simulink model "bldc_sixstep_f28069mLaunchPad"  (R2023b)
settings: Solver=FixedStepAuto  StartTime=0.0  StopTime=1.6  RelTol=1e-3  EnableMultiTasking=on
values from neighbouring files (symbols this model uses):
  bldc = mcb_SetPMSMMotorParameters('Teknic2310P')    [bldc_sixstep_f28069mLaunchPad_data.m]
  inverter = mcb_SetInverterParameters('BoostXL-DRV8305')    [bldc_sixstep_f28069mLaunchPad_data.m]
  PI_params = mcb_SetControllerParameters(bldc,inverter,PU_System,T_pwm,2*Ts,Ts_speed)    [bldc_sixstep_f28069mLaunchPad_data.m]
  PWM_frequency = 20e3    (= 20000)    [bldc_sixstep_f28069mLaunchPad_data.m]
  target = mcb_SetProcessorDetails('F28069M',PWM_frequency)    [bldc_sixstep_f28069mLaunchPad_data.m]
  Ts = T_pwm    (= 5e-05)    [bldc_sixstep_f28069mLaunchPad_data.m]
  Ts_motor_simscape = T_pwm/100    (= 5e-07)    [bldc_sixstep_f28069mLaunchPad_data.m]
  Ts_simulink = T_pwm/2    (= 2.5e-05)    [bldc_sixstep_f28069mLaunchPad_data.m]
  Ts_speed = 10*Ts    (= 0.0005)    [bldc_sixstep_f28069mLaunchPad_data.m]
libraries: nesl_utility x14, fl_lib x9, pil_lib x6, mcbcontrolslib x5, simulink x5, ee_lib x5, slpidlib x3, mcbpositiondecoderlib x2
(part 2 of 2)

== system bldc_sixstep_f28069mLaunchPad/Controller/Speed Control1/PI_Controller_Speed ==
  N_ref : Inport
  N_fb : Inport  Port=2
  Constant : Constant
  Discrete PI Controller with anti-windup & reset : slpidlib/PID Controller  Controller=PI  Form=Parallel  TimeDomain=Discrete-time  UseExternalTs=off  SampleTime=-1  IntegratorMethod=Forward Euler  FilterMethod=Forward Euler  ControllerParametersSource=external  P=1  I=1  UseKiTs=on  D=0  N=100  UseFilter=on  TunerSelectOption=Transfer Function Based (PID Tuner App)  InitialConditionSource=external  InitialConditionForIntegrator=0  InitialConditionForFilter=0  DifferentiatorICPrevScaledInput=0  ExternalReset=level  TrackingMode=off  Kt=1  LimitOutput=on  SatLimitsSource=internal  UpperSaturationLimit=1  LowerSaturationLimit=-1  LinearizeAsGain=on  AntiWindupMode=clamping  Kb=1  LimitIntegrator=off  UpperIntegratorSaturationLimit=inf  LowerIntegratorSaturationLimit=-inf  RndMeth=Simplest  POutMin=[]  POutMax=[]  IOutMin=[]  IOutMax=[]  DOutMin=[]  DOutMax=[]  NOutMin=[]  NOutMax=[]  SumOutMin=[]  SumOutMax=[]  SaturationOutDataTypeStr=Inherit: Inherit via back propagation  SaturationOutMin=[]  SaturationOutMax=[]  PParamMin=[]  PParamMax=[]  IParamMin=[]  IParamMax=[]  DParamMin=[]  DParamMax=[]  NParamMin=[]  NParamMax=[]  KbParamMin=[]  KbParamMax=[]  KtParamMin=[]  KtParamMax=[]  KbOutMin=[]  KbOutMax=[]  KtOutMin=[]  KtOutMax=[]  IntegratorOutMin=[]  IntegratorOutMax=[]  FilterOutMin=[]  FilterOutMax=[]  SumI1OutMin=[]  SumI1OutMax=[]  SumI2OutMin=[]  SumI2OutMax=[]  SumI3OutMin=[]  SumI3OutMax=[]  SumI4OutMin=[]  SumI4OutMax=[]  SumDOutMin=[]  SumDOutMax=[]  DifferentiatorOutMin=[]  DifferentiatorOutMax=[]  FilterDiffOutCoefMin=[]  FilterDiffOutCoefMax=[]  ReciprocalOutMin=[]  ReciprocalOutMax=[]  SumDenOutMin=[]  SumDenOutMax=[]  SumNumOutMin=[]  SumNumOutMax=[]  DivideOutMin=[]  DivideOutMax=[]  UdiffTsProdOutMin=[]  UdiffTsProdOutMax=[]  NTsProdOutMin=[]  NTsProdOutMax=[]  UintegralTsProdOutMin=[]  UintegralTsProdOutMax=[]  UngainTsProdOutMin=[]  UngainTsProdOutMax=[]  ClampingZeroOutDataTypeStr=Inherit: Inherit via back propagation  ClampingZeroOutMin=[]  ClampingZeroOutMax=[]  FilterDenConstantOutDataTypeStr=Inherit: Inherit via back propagation  FilterDenConstantOutMin=[]  FilterDenConstantOutMax=[]  PCopyOutDataTypeStr=Inherit: Inherit via back propagation  PCopyOutMin=[]  PCopyOutMax=[]  NCopyOutDataTypeStr=Inherit: Inherit via back propagation  NCopyOutMin=[]  NCopyOutMax=[]  IntegratorContinuousStateAttributes=''  IntegratorStateMustResolveToSignalObject=off  IntegratorRTWStateStorageClass=Auto  FilterContinuousStateAttributes=''  FilterStateMustResolveToSignalObject=off  FilterRTWStateStorageClass=Auto  ParallelPVariant=ExternalParameters  IdealPVariant=Disabled  IVariant=ExternalParameters  DVariant=Disabled  IntegratorVariant=Discrete  SatVariant=Enabled  AWVariant=DiscClampingParallel  PCopyVariant=Disabled  TRVariant=Disabled  FdbkBlocksVariant=Forward  IdealPFdbkVariant=Disabled  SatFdbkVariant=Disabled  DerivativeFilterVariant=Disabled  NVariant=Disabled  NCopyVariant=Disabled_SignalSpec  FilterICVariant=Disabled  IntegratorICVariant=ExternalICs  ExternalResetVariant=ExternalReset  TRSumVariant=Passthrough  SumFdbkVariant=Disabled  SumVariant=Sum_PI  TsampFilterVariant=InternalTs  TsampNgainVariant=Passthrough  TsampIntegralVariant=Disabled_SignalSpec  ExternalSaturationOutDataTypeStr=Inherit: Same as second input
      settings: LibrarySourceBlock=mcbcontrolslib/PI Controller
  Ki1 : Constant  Value=PI_params.Ki_speed*Ts_speed  OutDataTypeStr=dataType  SampleTime=-1
  Ki2 : Constant  Value=0  OutDataTypeStr=dataType  SampleTime=-1
  Kp1 : Constant  Value=PI_params.Kp_speed  OutDataTypeStr=dataType  SampleTime=-1
  Logical Operator : Logic  Operator=NOT  IconShape=distinctive  AllPortsSameDT=off  OutDataTypeStr=boolean
  Sum : Sum  Inputs=|+-  RndMeth=Round
  Zero_Cancellation : mcbcontrolslib/IIR Filter  VariantControl=Low Pass Filter  VariantSelect=Low-pass  Filter_constant=0.01*(Ts_speed/Ts)  advancedSettings=off  Ts=50e-6  cutOff_freq=353.6777
  Idc_ref : Outport  VectorParamsAs1DForOutWhenUnconnected=off
  wires:
  Discrete PI Controller with anti-windup & reset/1 -> Idc_ref/1
  Ki1/1 -> Discrete PI Controller with anti-windup & reset/3
  Kp1/1 -> Discrete PI Controller with anti-windup & reset/2
  N_fb/1 -> Sum/2
  N_ref/1 -> Zero_Cancellation/1
  Logical Operator/1 -> Discrete PI Controller with anti-windup & reset/4
  Ki2/1 -> Discrete PI Controller with anti-windup & reset/5
  Sum/1 -> Discrete PI Controller with anti-windup & reset/1
  Constant/1 -> Logical Operator/1
  Zero_Cancellation/1 -> Sum/1

== system bldc_sixstep_f28069mLaunchPad/Controller/Speed Control1/Speed_Ref_Selector ==
  Speed_Ref_In : Inport
  Speed_Ref_Open : Inport  Port=2
  Constant : Constant
  Switch : Switch  Criteria=u2 > Threshold  Threshold=0.5  SaturateOnIntegerOverflow=off  InputSameDT=off
  Speed_Ref_PU : Outport
  wires:
  Switch/1 -> Speed_Ref_PU/1
  Constant/1 -> Switch/2
  Speed_Ref_Open/1 -> Switch/3
  Speed_Ref_In/1 -> Switch/1

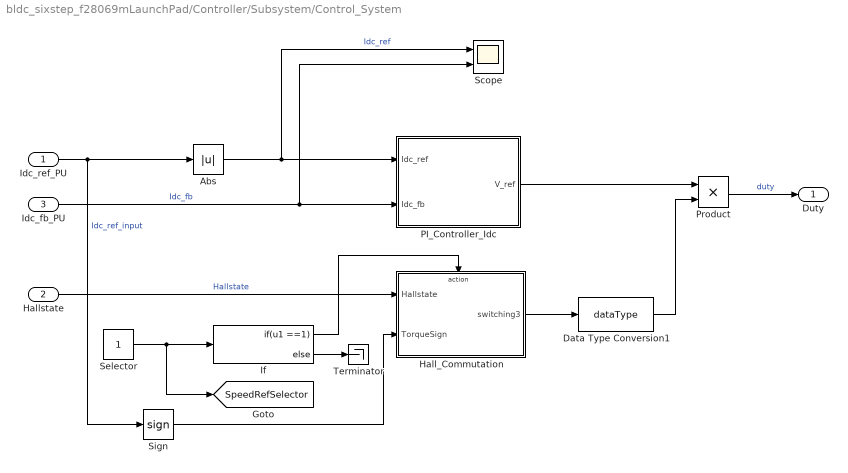
== system bldc_sixstep_f28069mLaunchPad/Controller/Subsystem/Control_System ==
  Idc_ref_PU : Inport
  Hallstate : Inport  Port=2
  Idc_fb_PU : Inport  Port=3
  Abs : Abs  SaturateOnIntegerOverflow=off
  Data Type Conversion1 : DataTypeConversion  OutDataTypeStr=dataType  RndMeth=Simplest  SaturateOnIntegerOverflow=off
  Hall_Commutation : Subsystem
  If : If  IfExpression=u1 ==1
  PI_Controller_Idc : Subsystem
  Product : Product  RndMeth=Simplest  OutDataTypeStr=Inherit: Same as first input
  Scope : Scope  NumInputPorts=2
  Selector : Constant  OutDataTypeStr=uint16  SampleTime=-1
  Sign : Signum
  Terminator : Terminator
  Duty : Outport  VectorParamsAs1DForOutWhenUnconnected=off
  tag scope: SpeedRefSelector=global
  wires:
  Hallstate/1 -> Hall_Commutation/1(Hallstate)  "Hallstate"
  If/1 -> Hall_Commutation/Action
  Idc_fb_PU/1 -> Scope/2, PI_Controller_Idc/2(Idc_fb)  "Idc_fb"
  Abs/1 -> Scope/1, PI_Controller_Idc/1(Idc_ref)  "Idc_ref"
  PI_Controller_Idc/1(V_ref) -> Product/1
  Idc_ref_PU/1 -> Sign/1, Abs/1  "Idc_ref_input"
  Product/1 -> Duty/1  "duty"
  Selector/1 -> If/1, [SpeedRefSelector]
  Sign/1 -> Hall_Commutation/2(TorqueSign)
  Data Type Conversion1/1 -> Product/2
  Hall_Commutation/1(switching3) -> Data Type Conversion1/1
  If/2 -> Terminator/1

== system bldc_sixstep_f28069mLaunchPad/Controller/Subsystem/Input scaling ==
  Iabc_meas_ADC : Inport
  Hall_Meas : Inport  Port=2
  Convert ADC value to PU : Subsystem
  Hall Feedback : Subsystem  TreatAsAtomicUnit=on
  Hall selected : Constant
  If : If  IfExpression=u1 ==1
  Terminator : Terminator
  Terminator1 : Terminator
  speed_PU : Outport  InitialOutput=0  VectorParamsAs1DForOutWhenUnconnected=off
  HallState : Outport  Port=2  InitialOutput=0  VectorParamsAs1DForOutWhenUnconnected=off
  Idc_meas_PU : Outport  Port=3
  wires:
  Hall Feedback/1(HallState) -> HallState/1
  Hall_Meas/1 -> Hall Feedback/1(Hall_Meas)
  If/1 -> Hall Feedback/Action
  Hall selected/1 -> If/1
  Hall Feedback/2(Speed_PU) -> speed_PU/1
  If/2 -> Terminator/1
  Iabc_meas_ADC/1 -> Convert ADC value to PU/1(Iabc_meas_ADC)
  Convert ADC value to PU/1(Idc_meas_PU) -> Idc_meas_PU/1
  Convert ADC value to PU/2(Ia_meas_PU) -> Terminator1/1

== system bldc_sixstep_f28069mLaunchPad/Controller/Subsystem/Inverter ==
  Inverter Signals : Inport
  Constant : Constant
  Data Type Duplicate : DataTypeDuplicate
  Switch : Switch  Threshold=0.5  RndMeth=Simplest  SaturateOnIntegerOverflow=off  InputSameDT=off
  stop : Constant  Value=[0 0 0 0 0 0]  OutDataTypeStr=Inherit: Inherit via back propagation
  Duty : Outport  VectorParamsAs1DForOutWhenUnconnected=off
  wires:
  Constant/1 -> Switch/2
  Switch/1 -> Duty/1
  Inverter Signals/1 -> Switch/1, Data Type Duplicate/1  "PWM Duty Cycles"
  stop/1 -> Switch/3, Data Type Duplicate/2

== system bldc_sixstep_f28069mLaunchPad/Controller/Subsystem/Sensor Driver Block ==
  fb_sim : Inport
  Bus Selector : BusSelector  OutputSignals=Iabc_fb,Hall_fb
  Iabc_Meas_ADC : Outport
  Hall_Meas : Outport  Port=2
  wires:
  Bus Selector/1 -> Iabc_Meas_ADC/1  "<Iabc_fb>"
  fb_sim/1 -> Bus Selector/1
  Bus Selector/2 -> Hall_Meas/1  "<Hall_fb>"

== system bldc_sixstep_f28069mLaunchPad/Controller - SIL/Subsystem/__InputSSForSFun__ ==
  Speed_ref_PU : Inport
  fb_sim : Inport  Port=2
  temporaryBusSelectName_1 : BusSelector  OutputSignals=Iabc_fb,Hall_fb
  __UniqueOutportName__1__ : Outport
  __UniqueOutportName__2__ : Outport  Port=2
  __UniqueOutportName__3__ : Outport  Port=3
  wires:
  temporaryBusSelectName_1/2 -> __UniqueOutportName__3__/1  "<Hall_fb>"
  temporaryBusSelectName_1/1 -> __UniqueOutportName__2__/1  "<Iabc_fb>"
  Speed_ref_PU/1 -> __UniqueOutportName__1__/1
  fb_sim/1 -> temporaryBusSelectName_1/1

== system bldc_sixstep_f28069mLaunchPad/Controller - SIL/Subsystem/__OutputSSForSFun__ ==
  __UniqueInportName__1__ : Inport
  Duty cycles : Outport
  wires:
  __UniqueInportName__1__/1 -> Duty cycles/1

== system bldc_sixstep_f28069mLaunchPad/Current control - SIL/Current control - SIL/__InputSSForSFun__ ==
  Idc_ref_PU : Inport
  fb_sim : Inport  Port=2
  temporaryBusSelectName_1 : BusSelector  OutputSignals=Iabc_fb,Hall_fb
  __UniqueOutportName__1__ : Outport
  __UniqueOutportName__2__ : Outport  Port=2
  __UniqueOutportName__3__ : Outport  Port=3
  wires:
  temporaryBusSelectName_1/2 -> __UniqueOutportName__3__/1  "<Hall_fb>"
  temporaryBusSelectName_1/1 -> __UniqueOutportName__2__/1  "<Iabc_fb>"
  Idc_ref_PU/1 -> __UniqueOutportName__1__/1
  fb_sim/1 -> temporaryBusSelectName_1/1

== system bldc_sixstep_f28069mLaunchPad/Current control - SIL/Current control - SIL/__OutputSSForSFun__ ==
  __UniqueInportName__1__ : Inport
  __UniqueInportName__2__ : Inport  Port=2
  Duty cycles : Outport
  Speed_fb_PU : Outport  Port=2
  wires:
  __UniqueInportName__2__/1 -> Speed_fb_PU/1
  __UniqueInportName__1__/1 -> Duty cycles/1

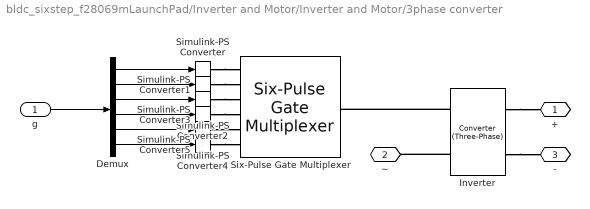
== system bldc_sixstep_f28069mLaunchPad/Inverter and Motor/Inverter and Motor/3phase converter ==
  g : Inport
  Demux : Demux  Outputs=6
  Inverter : ee_lib/Semiconductors & Converters/Converters/Converter (Three-Phase)  port_option=ee.enum.threePhasePort.composite  device_type=ee.enum.converters.switchingdevice.mosfet  K=0  Vf=0.8 V  Ron=0.001 Ohm  Rds=inverter.Rds_on Ohm  Goff=1e-5 1/Ohm  Vgt=1 V  Vgt_off=-1 V  Ih=1 A  Vth=0.7 V  diode_param=ee.enum.converters.protectiondiode.nodynamics  diode_Vf=0.7 V  diode_Ron=inverter.Rds_on Ohm  diode_Goff=1e-5 1/Ohm  diode_C=50 nF  diode_iRM=-235 A  diode_iF=300 A  diode_idot=-50 A/us  diode_trr_param=ee.enum.converters.diodetrr.trr_factor  diode_trr_factor=3  diode_trr=15 us  diode_Qrr=1.5e+3 s*uA  snubber_type=ee.enum.converters.snubber.exclude  Cs=1e-7 F  Rs=0.1 Ohm
  Simulink-PS Converter{,1..5} (6 alike) : nesl_utility/Simulink-PS Converter  PhysicalDomain=network_engine_domain  SubClassName=ps_input  LeftPortType=input  RightPortType=output  PseudoPeriodic=off  Frequencies=[]  NoiseDistribution=none  NoiseParameters=[]  Unit=1  AffineConversion=off  FilteringAndDerivatives=provide  SimscapeFilterOrder=1  InputFilterTimeConstant=0.001  UdotUserProvided=0
  Six-Pulse Gate Multiplexer : ee_lib/Semiconductors & Converters/Converters/Six-Pulse Gate Multiplexer  port_option=ee.enum.controlport.ps
  + : PMIOPort  Side=Right
  ~ : PMIOPort  Port=2  Side=Left
  - : PMIOPort  Port=3  Side=Right
  wires:
  g/1 -> Demux/1
  Demux/1 -> Simulink-PS Converter/1
  Demux/2 -> Simulink-PS Converter1/1
  Demux/3 -> Simulink-PS Converter2/1
  Demux/4 -> Simulink-PS Converter3/1
  Demux/6 -> Simulink-PS Converter5/1
  Demux/5 -> Simulink-PS Converter4/1
  connections:
  Simulink-PS Converter/RConn1 -- Six-Pulse Gate Multiplexer/LConn1
  Inverter/RConn2 -- -/RConn1
  Inverter/RConn1 -- +/RConn1
  Inverter/LConn2 -- ~/RConn1
  Inverter/LConn1 -- Six-Pulse Gate Multiplexer/RConn1
  Simulink-PS Converter1/RConn1 -- Six-Pulse Gate Multiplexer/LConn2
  Simulink-PS Converter2/RConn1 -- Six-Pulse Gate Multiplexer/LConn3
  Simulink-PS Converter3/RConn1 -- Six-Pulse Gate Multiplexer/LConn4
  Simulink-PS Converter4/RConn1 -- Six-Pulse Gate Multiplexer/LConn5
  Simulink-PS Converter5/RConn1 -- Six-Pulse Gate Multiplexer/LConn6

== system bldc_sixstep_f28069mLaunchPad/Inverter and Motor/Inverter and Motor/6-pulse PWM generator ==
  ModWave : Inport
  Relay : Relay
  Repeating Sequence Interpolated : simulink/Sources/Repeating Sequence Interpolated  OutValues="[0 1   0].'"  TimeValues=0.25/fs*[0 2 4].'  LookUpMeth=Interpolation-Use End Values  tsamp=Ts_motor_simscape  OutMin=[]  OutMax=[]  OutDataTypeStr=double  OutputDataTypeScalingMode=double  OutDataType=fixdt(0,8)  OutScaling=2^-10
  Sum : Sum  Inputs=|+-
  g : Outport
  wires:
  Relay/1 -> g/1
  Repeating Sequence Interpolated/1 -> Sum/2  "carrier"
  Sum/1 -> Relay/1
  ModWave/1 -> Sum/1

== system bldc_sixstep_f28069mLaunchPad/Inverter and Motor/Inverter and Motor/Scale ==
  duty_abc : Inport
  Constant : Constant  Value=0  OutDataTypeStr=single  SampleTime=Ts_motor_simscape
  Data Type Conversion : DataTypeConversion  SaturateOnIntegerOverflow=off  RndMeth=Floor
  Gain : Gain
  Rate Transition : RateTransition
  Sum : Sum  Inputs=|++
  ModWave : Outport
  wires:
  Gain/1 -> Data Type Conversion/1
  Data Type Conversion/1 -> Rate Transition/1
  Rate Transition/1 -> ModWave/1  "ModWave"
  duty_abc/1 -> Sum/1  "beforeGain"
  Constant/1 -> Sum/2
  Sum/1 -> Gain/1

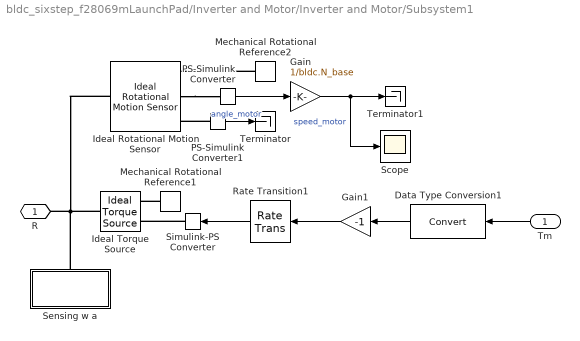
== system bldc_sixstep_f28069mLaunchPad/Inverter and Motor/Inverter and Motor/Subsystem1 ==
  Tm : Inport
  Data Type Conversion1 : DataTypeConversion  SaturateOnIntegerOverflow=off  RndMeth=Floor
  Gain : Gain  Gain=1/bldc.N_base
  Gain1 : Gain  Gain=-1
  Ideal Rotational Motion Sensor : fl_lib/Mechanical/Mechanical Sensors/Ideal Rotational Motion Sensor  reference=foundation.enum.MeasurementReference.difference  acceleration_port=false  velocity_port=true  position_port=true  wrap_angle=simscape.enum.onoff.off  offset=0 rad
  Ideal Torque Source : fl_lib/Mechanical/Mechanical Sources/Ideal Torque Source
  Mechanical Rotational Reference1 : fl_lib/Mechanical/Rotational Elements/Mechanical Rotational Reference
  Mechanical Rotational Reference2 : fl_lib/Mechanical/Rotational Elements/Mechanical Rotational Reference
  PS-Simulink Converter : nesl_utility/PS-Simulink Converter  PhysicalDomain=network_engine_domain  SubClassName=ps_output  LeftPortType=input  RightPortType=output  PseudoPeriodic=off  Frequencies=[]  VectorFormat=1-D array  Unit=rpm  AffineConversion=off
  PS-Simulink Converter1 : nesl_utility/PS-Simulink Converter  PhysicalDomain=network_engine_domain  SubClassName=ps_output  LeftPortType=input  RightPortType=output  PseudoPeriodic=off  Frequencies=[]  VectorFormat=1-D array  Unit=inherit  AffineConversion=off
  Rate Transition1 : RateTransition
  Scope : Scope
  Sensing w a : Subsystem
      mask Display: disp('w,Hall')
  Simulink-PS Converter : nesl_utility/Simulink-PS Converter  PhysicalDomain=network_engine_domain  SubClassName=ps_input  LeftPortType=input  RightPortType=output  PseudoPeriodic=off  Frequencies=[]  NoiseDistribution=none  NoiseParameters=[]  Unit=N*m  AffineConversion=off  FilteringAndDerivatives=provide  SimscapeFilterOrder=1  InputFilterTimeConstant=0.001  UdotUserProvided=0
  Terminator : Terminator
  Terminator1 : Terminator
  "R " : PMIOPort  Side=Right
  wires:
  Gain1/1 -> Rate Transition1/1
  Rate Transition1/1 -> Simulink-PS Converter/1
  Data Type Conversion1/1 -> Gain1/1
  Tm/1 -> Data Type Conversion1/1
  PS-Simulink Converter/1 -> Gain/1
  Gain/1 -> Scope/1, Terminator1/1  "speed_motor"
  PS-Simulink Converter1/1 -> Terminator/1  "angle_motor"
  connections:
  Mechanical Rotational Reference1/LConn1 -- Ideal Torque Source/RConn2
  Simulink-PS Converter/RConn1 -- Ideal Torque Source/RConn1
  Ideal Torque Source/LConn1 -- Sensing w a/LConn1 -- Ideal Rotational Motion Sensor/LConn1 -- "R "/RConn1
  Ideal Rotational Motion Sensor/RConn2 -- PS-Simulink Converter/LConn1
  PS-Simulink Converter1/LConn1 -- Ideal Rotational Motion Sensor/RConn3
  Mechanical Rotational Reference2/LConn1 -- Ideal Rotational Motion Sensor/RConn1

== system bldc_sixstep_f28069mLaunchPad/Inverter and Motor/Inverter and Motor/measVI ==
  Current Sensor (Three-Phase) : ee_lib/Sensors & Transducers/Current Sensor (Three-Phase)
  Line Voltage Sensor (Three-Phase) : ee_lib/Sensors & Transducers/Line Voltage Sensor (Three-Phase)
  PS-Simulink Converter2 : nesl_utility/PS-Simulink Converter  PhysicalDomain=network_engine_domain  SubClassName=ps_output  LeftPortType=input  RightPortType=output  PseudoPeriodic=off  Frequencies=[]  VectorFormat=1-D array  Unit=inherit  AffineConversion=off
  PS-Simulink Converter3 : nesl_utility/PS-Simulink Converter  PhysicalDomain=network_engine_domain  SubClassName=ps_output  LeftPortType=input  RightPortType=output  PseudoPeriodic=off  Frequencies=[]  VectorFormat=1-D array  Unit=inherit  AffineConversion=off
  ~1 From Inverter : PMIOPort  Side=Left
  ~2 to Motor : PMIOPort  Port=2  Side=Right
  tag scope: Iabc=global, Vabc=global
  wires:
  PS-Simulink Converter2/1 -> [Vabc]  "Vabc"
  PS-Simulink Converter3/1 -> [Iabc]  "Iabc"
  connections:
  Current Sensor (Three-Phase)/RConn1 -- PS-Simulink Converter3/LConn1
  PS-Simulink Converter2/LConn1 -- Line Voltage Sensor (Three-Phase)/RConn1
  Current Sensor (Three-Phase)/RConn2 -- ~2 to Motor/RConn1
  Line Voltage Sensor (Three-Phase)/LConn1 -- ~1 From Inverter/RConn1 -- Current Sensor (Three-Phase)/LConn1

== system bldc_sixstep_f28069mLaunchPad/Inverter and Motor/Sensor_Measurements/Halls ==
  x : Inport
  Demux : Demux  Outputs=3
  Gain : Gain  Gain=[4 2 1]  Multiplication=Matrix(K*u)
  Hall Signals HW : Subsystem
  Hall State Plant to HW : Subsystem
  Scope : Scope
  Scope1 : Scope  NumInputPorts=3
  Sum of Elements : Sum  Inputs=+
  y : Outport  VectorParamsAs1DForOutWhenUnconnected=off
  wires:
  Gain/1 -> Sum of Elements/1
  x/1 -> Gain/1
  Sum of Elements/1 -> Hall State Plant to HW/1(HallStatePlant)
  Hall State Plant to HW/1(HallstateHw) -> Scope/1, Hall Signals HW/1(HallState)  "HallState"
  Hall Signals HW/1(Hall Signals) -> Demux/1, y/1
  Demux/1 -> Scope1/1
  Demux/2 -> Scope1/2
  Demux/3 -> Scope1/3

== system bldc_sixstep_f28069mLaunchPad/Inverter and Motor/Sensor_Measurements/LowerSwitchCurrents ==
  In1 : Inport
  Constant : Constant  Value=0
  Switch : Switch  Criteria=u2 > Threshold  SaturateOnIntegerOverflow=off  InputSameDT=off
  cu : Outport
  wires:
  Constant/1 -> Switch/1
  In1/1 -> Switch/2, Switch/3
  Switch/1 -> cu/1  "cu"

== system bldc_sixstep_f28069mLaunchPad/Subsystem/Controller1/__InputSSForSFun__ ==
  Speed_ref : Inport
  fb_sim : Inport  Port=2
  temporaryBusSelectName_1 : BusSelector  OutputSignals=Iabc_fb,Hall_fb
  __UniqueOutportName__1__ : Outport
  __UniqueOutportName__2__ : Outport  Port=2
  __UniqueOutportName__3__ : Outport  Port=3
  wires:
  temporaryBusSelectName_1/2 -> __UniqueOutportName__3__/1  "<Hall_fb>"
  temporaryBusSelectName_1/1 -> __UniqueOutportName__2__/1  "<Iabc_fb>"
  Speed_ref/1 -> __UniqueOutportName__1__/1
  fb_sim/1 -> temporaryBusSelectName_1/1

== system bldc_sixstep_f28069mLaunchPad/Subsystem/Controller1/__OutputSSForSFun__ ==
  __UniqueInportName__1__ : Inport
  __UniqueInportName__2__ : Inport  Port=2
  __UniqueInportName__3__ : Inport  Port=3
  __UniqueInportName__4__ : Inport  Port=4
  __UniqueInportName__5__ : Inport  Port=5
  Speed ref : Outport
  Speed fb : Outport  Port=2
  Duty cycles : Outport  Port=3
  Idc ref : Outport  Port=4
  Idc_fb : Outport  Port=5
  wires:
  __UniqueInportName__5__/1 -> Idc_fb/1  "IDC"
  __UniqueInportName__4__/1 -> Idc ref/1
  __UniqueInportName__3__/1 -> Duty cycles/1
  __UniqueInportName__2__/1 -> Speed fb/1
  __UniqueInportName__1__/1 -> Speed ref/1

== system bldc_sixstep_f28069mLaunchPad/Controller/Subsystem/Control_System/Hall_Commutation ==
  Hallstate : Inport
  TorqueSign : Inport  Port=2
  Action Port : ActionPort  ActionPortLabel=if(u1 ==1)
  Six Step Commutation : mcbcontrolslib/Six Step Commutation  InputType=Hall  PositionUnit=Per unit  CommutationMode=120 deg  SequencePos=bldc.HallSequence  EnableCustomSwitching=off  CommutationSeqPos=[0 0 1 0 0 1;1 0 0 0 0 1;1 0 0 1 0 0;0 0 0 1 1 0;0 1 0 0 1 0;0 1 1 0 0 0]  CommutationSeqNeg="[0  1  1  0  0  0;0  1  0  0  1  0;0  0  0  1  1  0;1  0  0  1  0  0;1  0  0  0  0  1;0  0  1  0  0  1;]"
  switching3 : Outport
  wires:
  Hallstate/1 -> Six Step Commutation/1
  Six Step Commutation/1 -> switching3/1  "switching"
  TorqueSign/1 -> Six Step Commutation/2

== system bldc_sixstep_f28069mLaunchPad/Controller/Subsystem/Control_System/PI_Controller_Idc ==
  Idc_ref : Inport
  Idc_fb : Inport  Port=2
  Constant : Constant
  Discrete PI Controller with anti-windup & reset : slpidlib/PID Controller  Controller=PI  Form=Parallel  TimeDomain=Discrete-time  UseExternalTs=off  SampleTime=-1  IntegratorMethod=Forward Euler  FilterMethod=Forward Euler  ControllerParametersSource=external  P=1  I=1  UseKiTs=on  D=0  N=100  UseFilter=on  TunerSelectOption=Transfer Function Based (PID Tuner App)  InitialConditionSource=external  InitialConditionForIntegrator=0  InitialConditionForFilter=0  DifferentiatorICPrevScaledInput=0  ExternalReset=level  TrackingMode=off  Kt=1  LimitOutput=on  SatLimitsSource=internal  UpperSaturationLimit=1  LowerSaturationLimit=0  LinearizeAsGain=on  AntiWindupMode=clamping  Kb=1  LimitIntegrator=off  UpperIntegratorSaturationLimit=inf  LowerIntegratorSaturationLimit=-inf  RndMeth=Simplest  POutMin=[]  POutMax=[]  IOutMin=[]  IOutMax=[]  DOutMin=[]  DOutMax=[]  NOutMin=[]  NOutMax=[]  SumOutMin=[]  SumOutMax=[]  SaturationOutDataTypeStr=Inherit: Inherit via back propagation  SaturationOutMin=[]  SaturationOutMax=[]  PParamMin=[]  PParamMax=[]  IParamMin=[]  IParamMax=[]  DParamMin=[]  DParamMax=[]  NParamMin=[]  NParamMax=[]  KbParamMin=[]  KbParamMax=[]  KtParamMin=[]  KtParamMax=[]  KbOutMin=[]  KbOutMax=[]  KtOutMin=[]  KtOutMax=[]  IntegratorOutMin=[]  IntegratorOutMax=[]  FilterOutMin=[]  FilterOutMax=[]  SumI1OutMin=[]  SumI1OutMax=[]  SumI2OutMin=[]  SumI2OutMax=[]  SumI3OutMin=[]  SumI3OutMax=[]  SumI4OutMin=[]  SumI4OutMax=[]  SumDOutMin=[]  SumDOutMax=[]  DifferentiatorOutMin=[]  DifferentiatorOutMax=[]  FilterDiffOutCoefMin=[]  FilterDiffOutCoefMax=[]  ReciprocalOutMin=[]  ReciprocalOutMax=[]  SumDenOutMin=[]  SumDenOutMax=[]  SumNumOutMin=[]  SumNumOutMax=[]  DivideOutMin=[]  DivideOutMax=[]  UdiffTsProdOutMin=[]  UdiffTsProdOutMax=[]  NTsProdOutMin=[]  NTsProdOutMax=[]  UintegralTsProdOutMin=[]  UintegralTsProdOutMax=[]  UngainTsProdOutMin=[]  UngainTsProdOutMax=[]  ClampingZeroOutDataTypeStr=Inherit: Inherit via back propagation  ClampingZeroOutMin=[]  ClampingZeroOutMax=[]  FilterDenConstantOutDataTypeStr=Inherit: Inherit via back propagation  FilterDenConstantOutMin=[]  FilterDenConstantOutMax=[]  PCopyOutDataTypeStr=Inherit: Inherit via back propagation  PCopyOutMin=[]  PCopyOutMax=[]  NCopyOutDataTypeStr=Inherit: Inherit via back propagation  NCopyOutMin=[]  NCopyOutMax=[]  IntegratorContinuousStateAttributes=''  IntegratorStateMustResolveToSignalObject=off  IntegratorRTWStateStorageClass=Auto  FilterContinuousStateAttributes=''  FilterStateMustResolveToSignalObject=off  FilterRTWStateStorageClass=Auto  ParallelPVariant=ExternalParameters  IdealPVariant=Disabled  IVariant=ExternalParameters  DVariant=Disabled  IntegratorVariant=Discrete  SatVariant=Enabled  AWVariant=DiscClampingParallel  PCopyVariant=Disabled  TRVariant=Disabled  FdbkBlocksVariant=Forward  IdealPFdbkVariant=Disabled  SatFdbkVariant=Disabled  DerivativeFilterVariant=Disabled  NVariant=Disabled  NCopyVariant=Disabled_SignalSpec  FilterICVariant=Disabled  IntegratorICVariant=ExternalICs  ExternalResetVariant=ExternalReset  TRSumVariant=Passthrough  SumFdbkVariant=Disabled  SumVariant=Sum_PI  TsampFilterVariant=InternalTs  TsampNgainVariant=Passthrough  TsampIntegralVariant=Disabled_SignalSpec  ExternalSaturationOutDataTypeStr=Inherit: Same as second input
      settings: LibrarySourceBlock=mcbcontrolslib/PI Controller
  Ki : Constant  Value=PI_params.Ki_i*Ts  OutDataTypeStr=dataType  SampleTime=-1
  Kp : Constant  Value=PI_params.Kp_i  OutDataTypeStr=dataType  SampleTime=-1
  Kp1 : Constant  Value=0  OutDataTypeStr=dataType  SampleTime=-1
  Logical Operator : Logic  Operator=NOT  IconShape=distinctive  AllPortsSameDT=off  OutDataTypeStr=boolean
  Sum : Sum  Inputs=|+-  OutDataTypeStr=Inherit: Same as first input
  V_ref : Outport  VectorParamsAs1DForOutWhenUnconnected=off
  wires:
  Discrete PI Controller with anti-windup & reset/1 -> V_ref/1
  Constant/1 -> Logical Operator/1
  Idc_fb/1 -> Sum/2
  Idc_ref/1 -> Sum/1
  Sum/1 -> Discrete PI Controller with anti-windup & reset/1
  Logical Operator/1 -> Discrete PI Controller with anti-windup & reset/4
  Kp1/1 -> Discrete PI Controller with anti-windup & reset/5
  Kp/1 -> Discrete PI Controller with anti-windup & reset/2
  Ki/1 -> Discrete PI Controller with anti-windup & reset/3

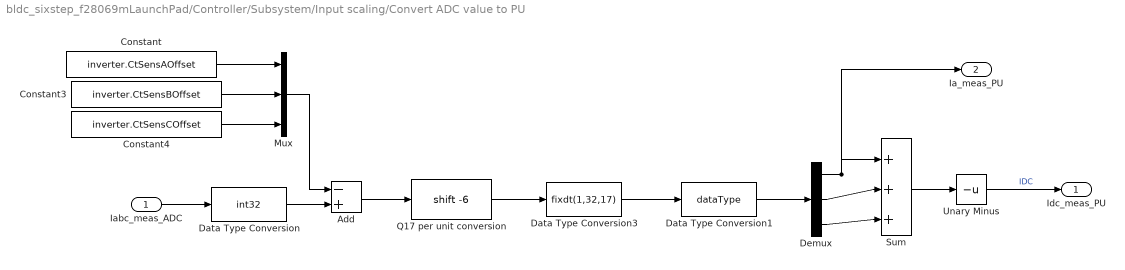
== system bldc_sixstep_f28069mLaunchPad/Controller/Subsystem/Input scaling/Convert ADC value to PU ==
  Iabc_meas_ADC : Inport
  Add : Sum  Inputs=-+
  Constant : Constant  Value=inverter.CtSensAOffset
  Constant3 : Constant  Value=inverter.CtSensBOffset
  Constant4 : Constant  Value=inverter.CtSensCOffset
  Data Type Conversion : DataTypeConversion  OutDataTypeStr=int32  ConvertRealWorld=Stored Integer (SI)  SaturateOnIntegerOverflow=off  RndMeth=Floor
  Data Type Conversion1 : DataTypeConversion  OutDataTypeStr=dataType  SaturateOnIntegerOverflow=off  RndMeth=Floor
  Data Type Conversion3 : DataTypeConversion  OutDataTypeStr=fixdt(1,32,17)  ConvertRealWorld=Stored Integer (SI)  RndMeth=Simplest  SaturateOnIntegerOverflow=off
  Demux : Demux  Outputs=3
  Mux : Mux  Inputs=3
  Q17 per unit conversion : ArithShift  BitShiftNumber=-6
  Sum : Sum  Inputs=|+++
  Unary Minus : UnaryMinus
  Idc_meas_PU : Outport
  Ia_meas_PU : Outport  Port=2  VectorParamsAs1DForOutWhenUnconnected=off
  wires:
  Data Type Conversion3/1 -> Data Type Conversion1/1
  Q17 per unit conversion/1 -> Data Type Conversion3/1
  Unary Minus/1 -> Idc_meas_PU/1  "IDC"
  Demux/2 -> Sum/2
  Demux/1 -> Sum/1, Ia_meas_PU/1
  Sum/1 -> Unary Minus/1
  Demux/3 -> Sum/3
  Data Type Conversion1/1 -> Demux/1
  Constant4/1 -> Mux/3
  Constant3/1 -> Mux/2
  Constant/1 -> Mux/1
  Iabc_meas_ADC/1 -> Data Type Conversion/1
  Data Type Conversion/1 -> Add/2
  Mux/1 -> Add/1
  Add/1 -> Q17 per unit conversion/1

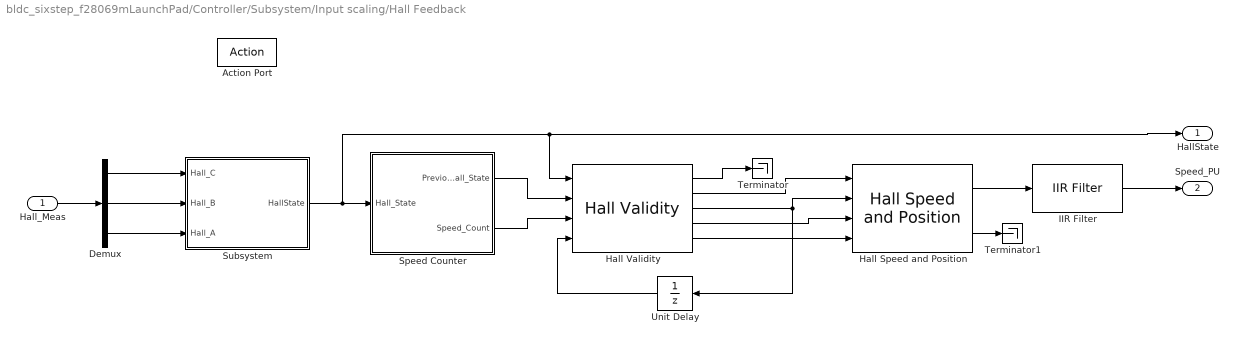
== system bldc_sixstep_f28069mLaunchPad/Controller/Subsystem/Input scaling/Hall Feedback ==
  Hall_Meas : Inport
  Action Port : ActionPort  ActionPortLabel=if(u1 ==1)
  Demux : Demux  Outputs=3
  Hall Speed and Position : mcbpositiondecoderlib/Hall Speed and Position  blkExecutionType=Speed  CounterSize=32 bits  ClkFreq=1/Ts  BlkSampleTime=Ts  PolePairs=bldc.p  MinSpeed=20  HallInterruptConfig=Every 60 Degrees  SpeedUnit=Per unit  PerUnitSpeed=PU_System.N_base  SpeedDataType=dataType  hallSequence=ABC  Sequence=[5,4,6,2,3,1]  EnableSecondOrder=1st Order  PositionUnit=Radians  PositionDataType=single
  Hall Validity : mcbpositiondecoderlib/Hall Validity  hallSequence=Custom sequence  sequence=bldc.HallSequence  CounterSize=32 bits
  IIR Filter : mcbcontrolslib/IIR Filter  VariantControl=Low Pass Filter  VariantSelect=Low-pass  Filter_constant=0.01  advancedSettings=off  Ts=50e-6  cutOff_freq=32.1525
  Speed Counter : Subsystem
  Subsystem : Subsystem
  Terminator : Terminator
  Terminator1 : Terminator
  Unit Delay : UnitDelay  InitialCondition=1  SampleTime=-1  HasFrameUpgradeWarning=on
  HallState : Outport  InitialOutput=0  VectorParamsAs1DForOutWhenUnconnected=off
  Speed_PU : Outport  Port=2  InitialOutput=0  VectorParamsAs1DForOutWhenUnconnected=off
  wires:
  Hall Speed and Position/1 -> IIR Filter/1
  Hall Speed and Position/2 -> Terminator1/1
  Hall Validity/2 -> Hall Speed and Position/1
  Hall Validity/3 -> Hall Speed and Position/2, Unit Delay/1
  Hall Validity/4 -> Hall Speed and Position/3
  Hall Validity/5 -> Hall Speed and Position/4
  Speed Counter/2(Speed_Count) -> Hall Validity/3
  Speed Counter/1(Previous_Hall_State) -> Hall Validity/2
  Subsystem/1(HallState) -> HallState/1, Hall Validity/1, Speed Counter/1(Hall_State)
  Unit Delay/1 -> Hall Validity/4
  Hall Validity/1 -> Terminator/1
  IIR Filter/1 -> Speed_PU/1
  Demux/1 -> Subsystem/1(Hall_C)
  Demux/2 -> Subsystem/2(Hall_B)
  Demux/3 -> Subsystem/3(Hall_A)
  Hall_Meas/1 -> Demux/1

== system bldc_sixstep_f28069mLaunchPad/Inverter and Motor/Inverter and Motor/Subsystem1/Sensing w a ==
  Hall sensor : Subsystem
  MRRef : fl_lib/Mechanical/Rotational Elements/Mechanical Rotational Reference
  Motion Sensor : fl_lib/Mechanical/Mechanical Sensors/Ideal Rotational Motion Sensor  reference=foundation.enum.MeasurementReference.difference  acceleration_port=false  velocity_port=true  position_port=true  wrap_angle=simscape.enum.onoff.off  offset=0 deg
  PS-Simulink Converter1 : nesl_utility/PS-Simulink Converter  PhysicalDomain=network_engine_domain  SubClassName=ps_output  LeftPortType=input  RightPortType=output  PseudoPeriodic=off  Frequencies=[]  VectorFormat=1-D array  Unit=rpm  AffineConversion=off
  PS-Simulink Converter2 : nesl_utility/PS-Simulink Converter  PhysicalDomain=network_engine_domain  SubClassName=ps_output  LeftPortType=input  RightPortType=output  PseudoPeriodic=off  Frequencies=[]  VectorFormat=1-D array  Unit=rad  AffineConversion=off
  Terminator : Terminator
  R : PMIOPort  Side=Left
  tag scope: HallSim=global
  wires:
  PS-Simulink Converter1/1 -> Terminator/1
  PS-Simulink Converter2/1 -> Hall sensor/1(theta)
  Hall sensor/1(Hall) -> [HallSim]
  connections:
  R/RConn1 -- Motion Sensor/LConn1
  Motion Sensor/RConn2 -- PS-Simulink Converter1/LConn1
  MRRef/LConn1 -- Motion Sensor/RConn1
  Motion Sensor/RConn3 -- PS-Simulink Converter2/LConn1

== system bldc_sixstep_f28069mLaunchPad/Inverter and Motor/Sensor_Measurements/Halls/Hall Signals HW ==
  HallState : Inport
  Bitwise AND1 : simulink/Logic and Bit Operations/Bitwise Operator  logicop=AND  UseBitMask=on  BitMask=bin2dec('00000010')  BitMaskRealWorld=Stored Integer
  Bitwise AND2 : simulink/Logic and Bit Operations/Bitwise Operator  logicop=AND  UseBitMask=on  BitMask=bin2dec('00000100')  BitMaskRealWorld=Stored Integer
  Bitwise AND3 : simulink/Logic and Bit Operations/Bitwise Operator  logicop=AND  UseBitMask=on  BitMask=bin2dec('00000001')  BitMaskRealWorld=Stored Integer
  Data Type Conversion : DataTypeConversion  OutDataTypeStr=boolean  SaturateOnIntegerOverflow=off  RndMeth=Floor
  Data Type Conversion1 : DataTypeConversion  OutDataTypeStr=boolean  SaturateOnIntegerOverflow=off  RndMeth=Floor
  Data Type Conversion2 : DataTypeConversion  OutDataTypeStr=boolean  SaturateOnIntegerOverflow=off  RndMeth=Floor
  Mux : Mux  Inputs=3
  Hall Signals : Outport
  wires:
  Mux/1 -> Hall Signals/1
  HallState/1 -> Bitwise AND3/1, Bitwise AND2/1, Bitwise AND1/1
  Data Type Conversion1/1 -> Mux/2
  Bitwise AND1/1 -> Data Type Conversion1/1
  Bitwise AND3/1 -> Data Type Conversion/1
  Bitwise AND2/1 -> Data Type Conversion2/1
  Data Type Conversion/1 -> Mux/3
  Data Type Conversion2/1 -> Mux/1

== system bldc_sixstep_f28069mLaunchPad/Inverter and Motor/Sensor_Measurements/Halls/Hall State Plant to HW ==
  HallStatePlant : Inport
  Data Type Conversion : DataTypeConversion  OutDataTypeStr=uint8  SaturateOnIntegerOverflow=off  RndMeth=Floor
  If Action Subsystem : Subsystem  TreatAsAtomicUnit=on
  If Action Subsystem1 : Subsystem  TreatAsAtomicUnit=on
  If Action Subsystem2 : Subsystem  TreatAsAtomicUnit=on
  If Action Subsystem3 : Subsystem  TreatAsAtomicUnit=on
  If Action Subsystem4 : Subsystem  TreatAsAtomicUnit=on
  If Action Subsystem5 : Subsystem  TreatAsAtomicUnit=on
  Merge : Merge  Inputs=6
  Switch Case : SwitchCase  CaseConditions={1,5,4,6,2,3}  ShowDefaultCase=off
  HallstateHw : Outport
  wires:
  Merge/1 -> Data Type Conversion/1
  HallStatePlant/1 -> Switch Case/1
  If Action Subsystem3/1(Out1) -> Merge/4
  Switch Case/4 -> If Action Subsystem3/Action
  If Action Subsystem5/1(Out1) -> Merge/6
  Switch Case/1 -> If Action Subsystem/Action
  Switch Case/6 -> If Action Subsystem5/Action
  Switch Case/3 -> If Action Subsystem2/Action
  If Action Subsystem/1(Out1) -> Merge/1
  If Action Subsystem4/1(Out1) -> Merge/5
  Switch Case/5 -> If Action Subsystem4/Action
  If Action Subsystem2/1(Out1) -> Merge/3
  If Action Subsystem1/1(Out1) -> Merge/2
  Switch Case/2 -> If Action Subsystem1/Action
  Data Type Conversion/1 -> HallstateHw/1

== system bldc_sixstep_f28069mLaunchPad/Controller/Subsystem/Input scaling/Hall Feedback/Speed Counter ==
  Hall_State : Inport
  AND : Logic  IconShape=distinctive  AllPortsSameDT=off  OutDataTypeStr=boolean
  Constant1 : Constant
  Constant4 : Constant  OutDataTypeStr=uint32  SampleTime=-1
  Delay : Delay  DelayLength=1  InitialCondition=1  ExternalReset=Level
      settings: InputPortMap=u0,r5
  Detect Change : simulink/Logic and Bit Operations/Detect Change  vinit=0  OutDataTypeStr=boolean
  Enabled Subsystem : Subsystem  TreatAsAtomicUnit=on
  Sum : Sum  Inputs=|++  OutDataTypeStr=uint32  AccumDataTypeStr=uint32  RndMeth=Simplest
  Unit Delay : UnitDelay  InitialCondition=1  SampleTime=-1  HasFrameUpgradeWarning=on
  Previous_Hall_State : Outport
  Speed_Count : Outport  Port=2
  wires:
  Delay/1 -> Unit Delay/1, Sum/2
  Constant4/1 -> Sum/1
  Sum/1 -> Delay/1
  Unit Delay/1 -> Enabled Subsystem/1(In1)
  Detect Change/1 -> Enabled Subsystem/Enable, AND/2
  Enabled Subsystem/1(Speed_Count) -> Speed_Count/1
  Hall_State/1 -> Enabled Subsystem/2(Hall_State), Detect Change/1
  Enabled Subsystem/2(PrevHallState) -> Previous_Hall_State/1
  AND/1 -> Delay/2
  Constant1/1 -> AND/1

== system bldc_sixstep_f28069mLaunchPad/Controller/Subsystem/Input scaling/Hall Feedback/Subsystem ==
  Hall_C : Inport
  Hall_B : Inport  Port=2
  Hall_A : Inport  Port=3
  Shift Arithmetic : ArithShift  BitShiftNumber=2  BitShiftDirection=Left
  Shift Arithmetic1 : ArithShift  BitShiftNumber=1  BitShiftDirection=Left
  Sum : Sum  Inputs=|+++
  HallState : Outport
  wires:
  Shift Arithmetic/1 -> Sum/1
  Shift Arithmetic1/1 -> Sum/2
  Hall_C/1 -> Shift Arithmetic/1
  Hall_A/1 -> Sum/3
  Sum/1 -> HallState/1
  Hall_B/1 -> Shift Arithmetic1/1

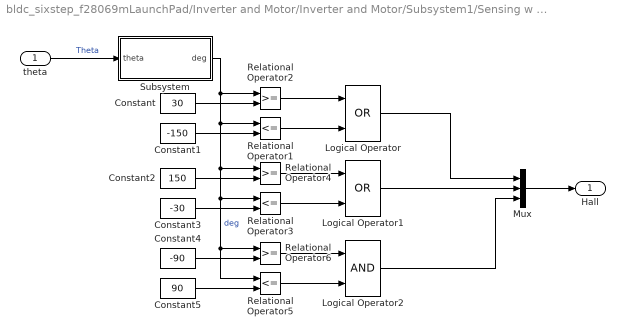
== system bldc_sixstep_f28069mLaunchPad/Inverter and Motor/Inverter and Motor/Subsystem1/Sensing w a/Hall sensor ==
  theta : Inport
  Constant : Constant  Value=30
  Constant1 : Constant  Value=-150
  Constant2 : Constant  Value=150
  Constant3 : Constant  Value=-30
  Constant4 : Constant  Value=-90
  Constant5 : Constant  Value=90
  Logical Operator : Logic  Operator=OR  AllPortsSameDT=off  OutDataTypeStr=boolean
  Logical Operator1 : Logic  Operator=OR  AllPortsSameDT=off  OutDataTypeStr=boolean
  Logical Operator2 : Logic  AllPortsSameDT=off  OutDataTypeStr=boolean
  Mux : Mux  Inputs=3
  Relational Operator1 : RelationalOperator  Operator=<=
  Relational Operator2 : RelationalOperator
  Relational Operator3 : RelationalOperator  Operator=<=
  Relational Operator4 : RelationalOperator
  Relational Operator5 : RelationalOperator  Operator=<=
  Relational Operator6 : RelationalOperator
  Subsystem : Subsystem
  Hall : Outport  VectorParamsAs1DForOutWhenUnconnected=off
  wires:
  theta/1 -> Subsystem/1(theta)  "Theta"
  Constant2/1 -> Relational Operator4/2
  Constant1/1 -> Relational Operator1/2
  Relational Operator4/1 -> Logical Operator1/1
  Constant/1 -> Relational Operator2/2
  Subsystem/1(deg) -> Relational Operator2/1, Relational Operator1/1, Relational Operator6/1, Relational Operator5/1, Relational Operator3/1, Relational Operator4/1  "deg"
  Relational Operator1/1 -> Logical Operator/2
  Relational Operator2/1 -> Logical Operator/1
  Mux/1 -> Hall/1
  Relational Operator3/1 -> Logical Operator1/2
  Constant5/1 -> Relational Operator5/2
  Constant4/1 -> Relational Operator6/2
  Relational Operator6/1 -> Logical Operator2/1
  Relational Operator5/1 -> Logical Operator2/2
  Logical Operator/1 -> Mux/1
  Logical Operator1/1 -> Mux/2
  Logical Operator2/1 -> Mux/3
  Constant3/1 -> Relational Operator3/2

== system bldc_sixstep_f28069mLaunchPad/Inverter and Motor/Sensor_Measurements/Halls/Hall State Plant to HW/If Action Subsystem ==
  Action Port : ActionPort  ActionPortLabel=case [ 1 ]:
  Constant : Constant  Value=bldc.HallSequence(1)  OutDataTypeStr=uint16
  Out1 : Outport
  wires:
  Constant/1 -> Out1/1

== system bldc_sixstep_f28069mLaunchPad/Inverter and Motor/Sensor_Measurements/Halls/Hall State Plant to HW/If Action Subsystem1 ==
  Action Port : ActionPort  ActionPortLabel=case [ 5 ]:
  Constant : Constant  Value=bldc.HallSequence(2)  OutDataTypeStr=uint16
  Out1 : Outport
  wires:
  Constant/1 -> Out1/1

== system bldc_sixstep_f28069mLaunchPad/Inverter and Motor/Sensor_Measurements/Halls/Hall State Plant to HW/If Action Subsystem2 ==
  Action Port : ActionPort  ActionPortLabel=case [ 4 ]:
  Constant : Constant  Value=bldc.HallSequence(3)  OutDataTypeStr=uint16
  Out1 : Outport
  wires:
  Constant/1 -> Out1/1

== system bldc_sixstep_f28069mLaunchPad/Inverter and Motor/Sensor_Measurements/Halls/Hall State Plant to HW/If Action Subsystem3 ==
  Action Port : ActionPort  ActionPortLabel=case [ 6 ]:
  Constant : Constant  Value=bldc.HallSequence(4)  OutDataTypeStr=uint16
  Out1 : Outport
  wires:
  Constant/1 -> Out1/1

== system bldc_sixstep_f28069mLaunchPad/Inverter and Motor/Sensor_Measurements/Halls/Hall State Plant to HW/If Action Subsystem4 ==
  Action Port : ActionPort  ActionPortLabel=case [ 2 ]:
  Constant : Constant  Value=bldc.HallSequence(5)  OutDataTypeStr=uint16
  Out1 : Outport
  wires:
  Constant/1 -> Out1/1

== system bldc_sixstep_f28069mLaunchPad/Inverter and Motor/Sensor_Measurements/Halls/Hall State Plant to HW/If Action Subsystem5 ==
  Action Port : ActionPort  ActionPortLabel=case [ 3 ]:
  Constant : Constant  Value=bldc.HallSequence(6)  OutDataTypeStr=uint16
  Out1 : Outport
  wires:
  Constant/1 -> Out1/1

== system bldc_sixstep_f28069mLaunchPad/Controller/Subsystem/Input scaling/Hall Feedback/Speed Counter/Enabled Subsystem ==
  In1 : Inport
  Hall_State : Inport  Port=2
  Enable : EnablePort
  Constant4 : Constant  OutDataTypeStr=uint32  SampleTime=-1
  Sum : Sum  Inputs=|++  OutDataTypeStr=uint32  AccumDataTypeStr=uint32  RndMeth=Simplest
  Unit Delay1 : UnitDelay  InitialCondition=1  SampleTime=-1  HasFrameUpgradeWarning=on
  Speed_Count : Outport
  PrevHallState : Outport  Port=2
  wires:
  Sum/1 -> Speed_Count/1
  Constant4/1 -> Sum/2
  In1/1 -> Sum/1
  Hall_State/1 -> Unit Delay1/1
  Unit Delay1/1 -> PrevHallState/1

== system bldc_sixstep_f28069mLaunchPad/Inverter and Motor/Inverter and Motor/Subsystem1/Sensing w a/Hall sensor/Subsystem ==
  theta : Inport
  Trigonometric Function : Trigonometry  Operator=sincos
  Trigonometric Function2 : Trigonometry  Operator=atan2
  mech->elec : Gain  Gain=bldc.p
  rad->deg : Gain  Gain=180/pi  SaturateOnIntegerOverflow=on  OutDataTypeStr=Inherit: Same as input  ParamDataTypeStr=Inherit: Same as input
  deg : Outport  VectorParamsAs1DForOutWhenUnconnected=off
  wires:
  mech->elec/1 -> Trigonometric Function/1
  Trigonometric Function/2 -> Trigonometric Function2/2
  rad->deg/1 -> deg/1
  theta/1 -> mech->elec/1
  Trigonometric Function/1 -> Trigonometric Function2/1
  Trigonometric Function2/1 -> rad->deg/1
